simulink model "Observer_e_modello"  (R2023a)
settings: Solver=ode45  StartTime=0.0  StopTime=102  RelTol=1e-2  EnableMultiTasking=on
values from neighbouring files (symbols this model uses):
  xk0_mod = 0.9*ones(states_tot, 1)    [Convergence_observer.m]
  xk0_obs = 0*ones(states_tot, 1)    [Convergence_observer.m]
  yk2_0 = 0.5*ones(4,1)    [Convergence_observer.m]
  yk6_0 = 0.5*ones(4,1)    [Convergence_observer.m]
undefined symbols (not defined in the file or in its folder): F0A, R1, R2, R3
settings Model: Creator=scattolini  LastModifiedBy=laura
settings SolverCC: AlgebraicLoopSolver=TrustRegion
settings DataIOCC: LimitDataPoints=on  SaveFormat=Array  SignalLoggingSaveFormat=ModelDataLogs  ReturnWorkspaceOutputs=off
settings OptimizationCC: BlockReduction=off  DefaultParameterBehavior=Inlined  InlineInvariantSignals=on  BufferReuse=off  ExpressionDepthLimit=2147483647  InitFltsAndDblsToZero=on  LifeSpan=inf
settings DebuggingCC: SaveWithParameterizedLinksMsg=none  UnderspecifiedInitializationDetection=Classic  MergeDetectMultiDrivingBlocksExec=none  SignalResolutionControl=TryResolveAllWithWarning  SolverPrmCheckMsg=warning  MultiTaskDSMMsg=warning  MultiTaskCondExecSysMsg=none  FcnCallInpInsideContextMsg=warning  UnconnectedInputMsg=warning  UnconnectedOutputMsg=warning  UnconnectedLineMsg=warning  StateNameClashWarn=warning  SFUnexpectedBacktrackingDiag=warning  SFNoUnconditionalDefaultTransitionDiag=warning  SFExecutionAtInitializationDiag=none  ArithmeticOperatorsInVariantConditions=warning
settings HardwareCC: ProdBitPerPointer=32  ProdBitPerSizeT=32  ProdBitPerPtrDiffT=32  ProdLargestAtomicFloat=None  ProdIntDivRoundTo=Undefined  ProdEndianess=Unspecified  ProdWordSize=32  ProdHWDeviceType=32-bit Generic
settings ModelReferenceCC: EnableRefExpFcnMdlSchedulingChecks=on  PropagateSignalLabelsOutOfModel=off
settings RTWCC: DLArmComputeVersion=19.05
settings CodeAppCC: StateflowObjectComments=on
settings GRTTargetCC: TargetFcnLib=ansi_tfl_tmw.mat  TargetLangStandard=C89/C90 (ANSI)  CombineOutputUpdateFcns=off  GRTInterface=on
settings ConfigComp: CovMetricSettings=dw  CovSaveCumulativeToWorkspaceVar=on  CovSaveSingleToWorkspaceVar=on

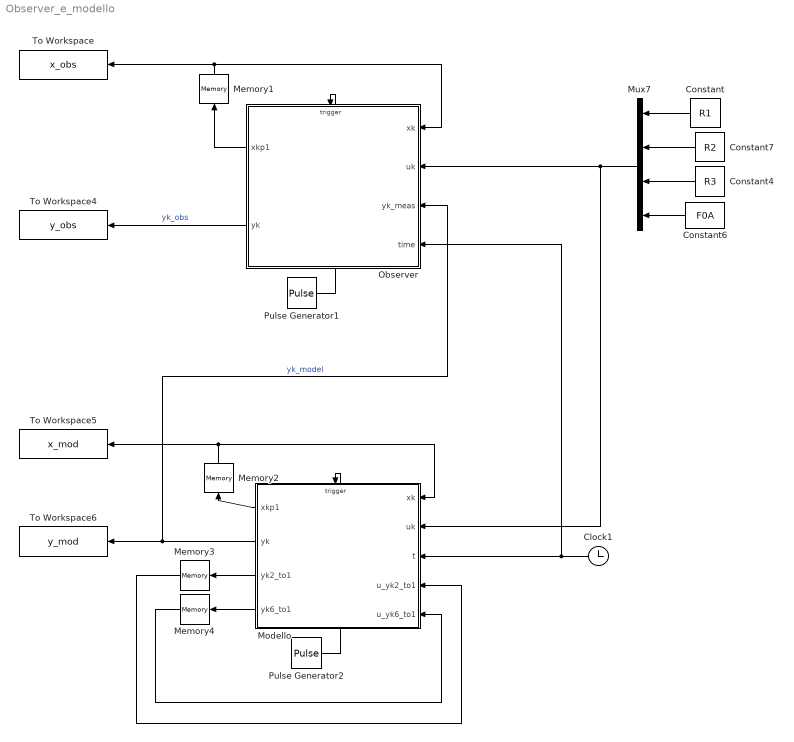
== system Observer_e_modello ==
  Clock1 : Clock
  Constant : Constant  Value=R1
  Constant4 : Constant  Value=R3
  Constant6 : Constant  Value=F0A
  Constant7 : Constant  Value=R2
  Memory1 : Memory  InitialCondition=xk0_obs
  Memory2 : Memory  InitialCondition=xk0_mod
  Memory3 : Memory  InitialCondition=yk2_0
  Memory4 : Memory  InitialCondition=yk6_0
  "Modello " : Subsystem  TreatAsAtomicUnit=on
  Mux7 : Mux
  Observer : Subsystem  TreatAsAtomicUnit=on
  Pulse Generator1 : DiscretePulseGenerator  PulseType=Time based  Period=1  PulseWidth=5
  Pulse Generator2 : DiscretePulseGenerator  PulseType=Time based  Period=1  PulseWidth=5
  To Workspace : ToWorkspace  VariableName=x_obs  SampleTime=1
  To Workspace4 : ToWorkspace  VariableName=y_obs  SampleTime=1
  To Workspace5 : ToWorkspace  VariableName=x_mod  SampleTime=1
  To Workspace6 : ToWorkspace  VariableName=y_mod  SampleTime=1
  wires:
  Pulse Generator1/1 -> Observer/Trigger
  Observer/1(xkp1) -> Memory1/1
  Memory1/1 -> Observer/1(xk), To Workspace/1
  Observer/2(yk) -> To Workspace4/1  "yk_obs"
  Mux7/1 -> Observer/2(uk), "Modello "/2(uk)
  Constant6/1 -> Mux7/4
  Clock1/1 -> Observer/4(time), "Modello "/3(t)
  "Modello "/1(xkp1) -> Memory2/1
  "Modello "/2(yk) -> Observer/3(yk_meas), To Workspace6/1  "yk_model"
  Memory2/1 -> "Modello "/1(xk), To Workspace5/1
  Pulse Generator2/1 -> "Modello "/Trigger
  "Modello "/3(yk2_to1) -> Memory3/1
  Memory3/1 -> "Modello "/4(u_yk2_to1)
  "Modello "/4(yk6_to1) -> Memory4/1
  Memory4/1 -> "Modello "/5(u_yk6_to1)
  Constant/1 -> Mux7/1
  Constant7/1 -> Mux7/2
  Constant4/1 -> Mux7/3

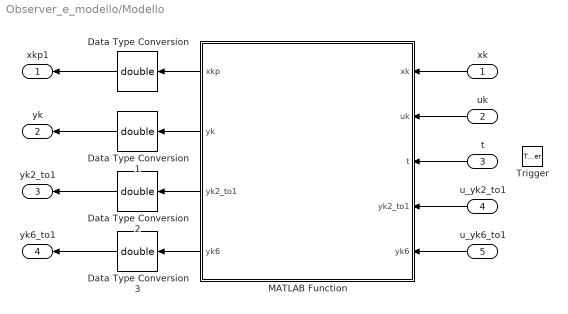
== system Observer_e_modello/Modello  ==
  xk : Inport
  uk : Inport  Port=2
  t : Inport  Port=3
  u_yk2_to1 : Inport  Port=4
  u_yk6_to1 : Inport  Port=5
  Trigger : TriggerPort  VariantControl=(inherit)
  Data Type Conversion{,1..3} (4 alike) : DataTypeConversion  OutDataTypeStr=double  RndMeth=Nearest  SaturateOnIntegerOverflow=off
  MATLAB Function : MATLAB Function  TreatAsAtomicUnit=on
  xkp1 : Outport
  yk : Outport  Port=2
  yk2_to1 : Outport  Port=3
  yk6_to1 : Outport  Port=4
  wires:
  xk/1 -> MATLAB Function/1(xk)
  MATLAB Function/2(yk) -> Data Type Conversion1/1
  MATLAB Function/1(xkp) -> Data Type Conversion/1
  Data Type Conversion/1 -> xkp1/1
  Data Type Conversion1/1 -> yk/1
  uk/1 -> MATLAB Function/2(uk)
  t/1 -> MATLAB Function/3(t)
  Data Type Conversion2/1 -> yk2_to1/1
  MATLAB Function/3(yk2_to1) -> Data Type Conversion2/1
  Data Type Conversion3/1 -> yk6_to1/1
  MATLAB Function/4(yk6) -> Data Type Conversion3/1
  u_yk6_to1/1 -> MATLAB Function/5("yk6 ")
  u_yk2_to1/1 -> MATLAB Function/4("yk2_to1 ")

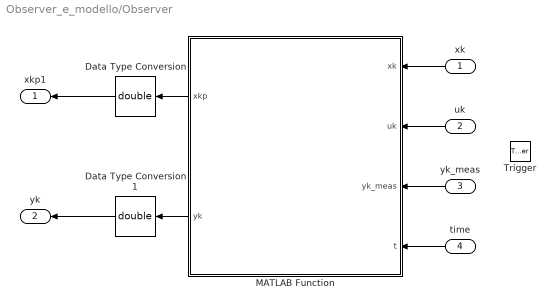
== system Observer_e_modello/Observer ==
  xk : Inport
  uk : Inport  Port=2
  yk_meas : Inport  Port=3
  time : Inport  Port=4
  Trigger : TriggerPort  VariantControl=(inherit)
  Data Type Conversion : DataTypeConversion  OutDataTypeStr=double  RndMeth=Nearest  SaturateOnIntegerOverflow=off
  Data Type Conversion1 : DataTypeConversion  OutDataTypeStr=double  RndMeth=Nearest  SaturateOnIntegerOverflow=off
  MATLAB Function : MATLAB Function  TreatAsAtomicUnit=on
  xkp1 : Outport
  yk : Outport  Port=2
  wires:
  xk/1 -> MATLAB Function/1(xk)
  uk/1 -> MATLAB Function/2(uk)
  MATLAB Function/2(yk) -> Data Type Conversion1/1
  MATLAB Function/1(xkp) -> Data Type Conversion/1
  Data Type Conversion/1 -> xkp1/1
  Data Type Conversion1/1 -> yk/1
  yk_meas/1 -> MATLAB Function/3(yk_meas)
  time/1 -> MATLAB Function/4(t)

== matlab function Observer_e_modello/Observer/MATLAB Function ==
  data: xkp output; xk input; uk input; yk_meas input; t input; yk output
function [xkp, yk] = RNN(xk, uk, yk_meas, t)

    if t <= 1
        xk = 0*ones(18, 1);
    end

    n_states = [3,3,3,3,3,3];
    layers_file = load("layers_file.mat");
    layers_file = layers_file.layers_file;
    input_scaler_bias = load("input_scaler_bias.mat");
    input_scaler_scale_common = load("input_scaler_scale_common.mat");
    output_scaler_bias = load("output_scaler_bias.mat");
    output_scaler_scale_common = load("output_scaler_scale_common.mat");
    
    % Best observer weight
    Lz1_sol = load("Lz1_sol.mat");
    Lf1_sol = load("Lf1_sol.mat");
    Lz1 = Lz1_sol.Lz1;
    Lf1 = Lf1_sol.Lf1;
    Lz2_sol = load("Lz2_sol.mat");
    Lf2_sol = load("Lf2_sol.mat");
    Lz2 = Lz2_sol.Lz2;
    Lf2 = Lf2_sol.Lf2;
    Lz3_sol = load("Lz3_sol.mat");
    Lf3_sol = load("Lf3_sol.mat");
    Lz3 = Lz3_sol.Lz3;
    Lf3 = Lf3_sol.Lf3;
    Lz4_sol = load("Lz4_sol.mat");
    Lf4_sol = load("Lf4_sol.mat");
    Lz4 = Lz4_sol.Lz4;
    Lf4 = Lf4_sol.Lf4;
    Lz5_sol = load("Lz5_sol.mat");
    Lf5_sol = load("Lf5_sol.mat");
    Lz5 = Lz5_sol.Lz5;
    Lf5 = Lf5_sol.Lf5;
    Lz6_sol = load("Lz6_sol.mat");
    Lf6_sol = load("Lf6_sol.mat");
    Lz6 = Lz6_sol.Lz6;
    Lf6 = Lf6_sol.Lf6;

    % Scale input and output
    uk = (uk  - (input_scaler_bias.input_scaler_bias).') ./ (input_scaler_scale_common.input_scaler_scale_common).';
    %yk_meas = [yk_meas(1)*yk_meas(2); yk_meas(1)*yk_meas(3); yk_meas(1)*yk_meas(4); yk_meas(1)*yk_meas(5); yk_meas(6)*yk_meas(7); yk_meas(6)*yk_meas(8); yk_meas(6)*yk_meas(9); yk_meas(6)*yk_meas(10); yk_meas(11)*yk_meas(12); yk_meas(11)*yk_meas(13); yk_meas(11)*yk_meas(14); yk_meas(11)*yk_meas(15); yk_meas(16)*yk_meas(17); yk_meas(11)*yk_meas(18); yk_meas(11)*yk_meas(19); yk_meas(11)*yk_meas(20); yk_meas(21)*yk_meas(22); yk_meas(21)*yk_meas(23); yk_meas(21)*yk_meas(24); yk_meas(21)*yk_meas(25); yk_meas(26)*yk_meas(27); yk_meas(26)*yk_meas(28); yk_meas(26)*yk_meas(29); yk_meas(26)*yk_meas(30); yk_meas(31)*yk_meas(32); yk_meas(31)*yk_meas(33); yk_meas(31)*yk_meas(34); yk_meas(31)*yk_meas(35)];
    yk_meas = (yk_meas  - (output_scaler_bias.output_scaler_bias).') ./ (output_scaler_scale_common.output_scaler_scale_common).';

    % GRU 1
    yk1_meas = yk_meas(1:4,:);
    yk2_to1_meas = yk_meas(5:8,:);
    yk6_meas = yk_meas(25:28,:);
    uk1 = [uk(1,:); uk(3:4,:); yk2_to1_meas; yk6_meas];
    xk1 = xk(1:n_states(1),:);    
    yk1 = layers_file.layers{1,2}.weights.weight * xk1 + (layers_file.layers{1,2}.weights.bias).';
    zk1 = sigmoidfunction((layers_file.layers{1,1}.weights.Wzf(:,1:n_states(1))).' * uk1 + (layers_file.layers{1,1}.weights.Uzf(:,1:n_states(1))).' * xk1 + (layers_file.layers{1,1}.weights.bzf(:,1:n_states(1))).' + Lz1*(yk1_meas-yk1) );
    fk1 = sigmoidfunction((layers_file.layers{1,1}.weights.Wzf(:,n_states(1)+1:end)).' * uk1 + (layers_file.layers{1,1}.weights.Uzf(:,n_states(1)+1:end)).' * xk1 + (layers_file.layers{1,1}.weights.bzf(:,n_states(1)+1:end)).' + Lf1*(yk1_meas-yk1) );
    phi1 = tanh((layers_file.layers{1,1}.weights.Wr).' * uk1 + (layers_file.layers{1,1}.weights.Ur).' * (fk1.* xk1) + (layers_file.layers{1,1}.weights.br).');
    xkp1 = zk1 .* xk1 + (1-zk1) .* phi1;
    
    % GRU 2    
    yk2_meas = yk_meas(5:12,:);
    yk2_to3_meas = yk_meas(9:12,:);
    uk2 = [uk(1,:); uk(3:4,:); yk1_meas];
    xk2 = xk(n_states(1)+1:n_states(1)+n_states(2),:);
    yk2 = layers_file.layers{1,4}.weights.weight * xk2 + (layers_file.layers{1,4}.weights.bias).';
    zk2 = sigmoidfunction((layers_file.layers{1,3}.weights.Wzf(:,1:n_states(2))).' * uk2 + (layers_file.layers{1,3}.weights.Uzf(:,1:n_states(2))).' * xk2 + (layers_file.layers{1,3}.weights.bzf(:,1:n_states(2))).' + Lz2*(yk2_meas-yk2) );
    fk2 = sigmoidfunction((layers_file.layers{1,3}.weights.Wzf(:,n_states(2)+1:end)).' * uk2 + (layers_file.layers{1,3}.weights.Uzf(:,n_states(2)+1:end)).' * xk2 + (layers_file.layers{1,3}.weights.bzf(:,n_states(2)+1:end)).' + Lf2*(yk2_meas-yk2) );
    phi2 = tanh((layers_file.layers{1,3}.weights.Wr).' * uk2 + (layers_file.layers{1,3}.weights.Ur).' * (fk2.* xk2) + (layers_file.layers{1,3}.weights.br).');
    xkp2 = zk2 .* xk2 + (1-zk2) .* phi2;
    
    % GRU 3
    yk3_meas = yk_meas(13:16,:);
    uk3 = [uk(2:4,:); yk2_to3_meas];
    xk3 = xk(n_states(1)+n_states(2)+1:n_states(1)+n_states(2)+n_states(3),:);
    yk3 = layers_file.layers{1,6}.weights.weight * xk3 + (layers_file.layers{1,6}.weights.bias).';
    zk3 = sigmoidfunction((layers_file.layers{1,5}.weights.Wzf(:,1:n_states(3))).' * uk3 + (layers_file.layers{1,5}.weights.Uzf(:,1:n_states(3))).' * xk3 + (layers_file.layers{1,5}.weights.bzf(:,1:n_states(3))).' + Lz3*(yk3_meas-yk3) );
    fk3 = sigmoidfunction((layers_file.layers{1,5}.weights.Wzf(:,n_states(3)+1:end)).' * uk3 + (layers_file.layers{1,5}.weights.Uzf(:,n_states(3)+1:end)).' * xk3 + (layers_file.layers{1,5}.weights.bzf(:,n_states(3)+1:end)).' + Lf3*(yk3_meas-yk3) );
    phi3 = tanh((layers_file.layers{1,5}.weights.Wr).' * uk3 + (layers_file.layers{1,5}.weights.Ur).' * (fk3.* xk3) + (layers_file.layers{1,5}.weights.br).');
    xkp3 = zk3 .* xk3 + (1-zk3) .* phi3;

    % GRU 4
    yk4_meas = yk_meas(17:20,:);
    uk4 = [uk(2:4,:); yk3_meas];
    xk4 = xk(n_states(1)+n_states(2)+n_states(3)+1:n_states(1)+n_states(2)+n_states(3)+n_states(4),:);
    yk4 = layers_file.layers{1,8}.weights.weight * xk4 + (layers_file.layers{1,8}.weights.bias).';
    zk4 = sigmoidfunction((layers_file.layers{1,7}.weights.Wzf(:,1:n_states(4))).' * uk4 + (layers_file.layers{1,7}.weights.Uzf(:,1:n_states(4))).' * xk4 + (layers_file.layers{1,7}.weights.bzf(:,1:n_states(4))).' + Lz4*(yk4_meas-yk4) );
    fk4 = sigmoidfunction((layers_file.layers{1,7}.weights.Wzf(:,n_states(4)+1:end)).' * uk4 + (layers_file.layers{1,7}.weights.Uzf(:,n_states(4)+1:end)).' * xk4 + (layers_file.layers{1,7}.weights.bzf(:,n_states(4)+1:end)).' + Lf4*(yk4_meas-yk4) );
    phi4 = tanh((layers_file.layers{1,7}.weights.Wr).' * uk4 + (layers_file.layers{1,7}.weights.Ur).' * (fk4.* xk4) + (layers_file.layers{1,7}.weights.br).');
    xkp4 = zk4 .* xk4 + (1-zk4) .* phi4;

    % GRU 5
    yk5_meas = yk_meas(21:24,:);
    uk5 = [uk(2:4,:); yk4_meas];
    xk5 = xk(n_states(1)+n_states(2)+n_states(3)+n_states(4)+1:n_states(1)+n_states(2)+n_states(3)+n_states(4)+n_states(5),:);
    yk5 = layers_file.layers{1,10}.weights.weight * xk5 + (layers_file.layers{1,10}.weights.bias).';
    zk5 = sigmoidfunction((layers_file.layers{1,9}.weights.Wzf(:,1:n_states(5))).' * uk5 + (layers_file.layers{1,9}.weights.Uzf(:,1:n_states(5))).' * xk5 + (layers_file.layers{1,9}.weights.bzf(:,1:n_states(5))).' + Lz5*(yk5_meas-yk5) );
    fk5 = sigmoidfunction((layers_file.layers{1,9}.weights.Wzf(:,n_states(5)+1:end)).' * uk5 + (layers_file.layers{1,9}.weights.Uzf(:,n_states(5)+1:end)).' * xk5 + (layers_file.layers{1,9}.weights.bzf(:,n_states(5)+1:end)).' + Lf5*(yk5_meas-yk5) );
    phi5 = tanh((layers_file.layers{1,9}.weights.Wr).' * uk5 + (layers_file.layers{1,9}.weights.Ur).' * (fk5.* xk5) + (layers_file.layers{1,9}.weights.br).');
    xkp5 = zk5 .* xk5 + (1-zk5) .* phi5;

    % GRU 6
    uk6 = [uk(2:4,:); yk5_meas];
    xk6 = xk(n_states(1)+n_states(2)+n_states(3)+n_states(4)+n_states(5)+1:n_states(1)+n_states(2)+n_states(3)+n_states(4)+n_states(5)+n_states(6),:);
    yk6 = layers_file.layers{1,12}.weights.weight * xk6 + (layers_file.layers{1,12}.weights.bias).';
    zk6 = sigmoidfunction((layers_file.layers{1,11}.weights.Wzf(:,1:n_states(6))).' * uk6 + (layers_file.layers{1,11}.weights.Uzf(:,1:n_states(6))).' * xk6 + (layers_file.layers{1,11}.weights.bzf(:,1:n_states(6))).' + Lz6*(yk6_meas-yk6) );
    fk6 = sigmoidfunction((layers_file.layers{1,11}.weights.Wzf(:,n_states(6)+1:end)).' * uk6 + (layers_file.layers{1,11}.weights.Uzf(:,n_states(6)+1:end)).' * xk6 + (layers_file.layers{1,11}.weights.bzf(:,n_states(6)+1:end)).' + Lf6*(yk6_meas-yk6) );
    phi6 = tanh((layers_file.layers{1,11}.weights.Wr).' * uk6 + (layers_file.layers{1,11}.weights.Ur).' * (fk6.* xk6) + (layers_file.layers{1,11}.weights.br).');
    xkp6 = zk6 .* xk6 + (1-zk6) .* phi6;
    
    % Overall
    xkp = [xkp1; xkp2; xkp3; xkp4; xkp5; xkp6];
    yk = [yk1; yk2; yk3; yk4; yk5; yk6];
    yk = yk .* (output_scaler_scale_common.output_scaler_scale_common).' + (output_scaler_bias.output_scaler_bias).';
end

== matlab function Observer_e_modello/Modello /MATLAB Function ==
  data: xkp output; xk input; uk input; t input; yk output; yk2_to1 output; yk6 output; yk2_to1 input; yk6 input
function [xkp, yk, yk2_to1, yk6] = RNN(xk, uk, t, yk2_to1, yk6)

    if t <= 1
        xk = 0.9*ones(18, 1);
    end

    n_states = [3,3,3,3,3,3];
    layers_file = load("layers_file.mat");
    layers_file = layers_file.layers_file;
    input_scaler_bias = load("input_scaler_bias.mat");
    input_scaler_scale_common = load("input_scaler_scale_common.mat");
    output_scaler_bias = load("output_scaler_bias.mat");
    output_scaler_scale_common = load("output_scaler_scale_common.mat");

    % Scale input and output
    uk = (uk  - (input_scaler_bias.input_scaler_bias).') ./ (input_scaler_scale_common.input_scaler_scale_common).';

    % GRU 1
    uk1 = [uk(1,:); uk(3:4,:); yk2_to1; yk6];
    xk1 = xk(1:n_states(1),:); 
    zk1 = sigmoidfunction((layers_file.layers{1,1}.weights.Wzf(:,1:n_states(1))).' * uk1 + (layers_file.layers{1,1}.weights.Uzf(:,1:n_states(1))).' * xk1 + (layers_file.layers{1,1}.weights.bzf(:,1:n_states(1))).');
    fk1 = sigmoidfunction((layers_file.layers{1,1}.weights.Wzf(:,n_states(1)+1:end)).' * uk1 + (layers_file.layers{1,1}.weights.Uzf(:,n_states(1)+1:end)).' * xk1 + (layers_file.layers{1,1}.weights.bzf(:,n_states(1)+1:end)).');
    phi1 = tanh((layers_file.layers{1,1}.weights.Wr).' * uk1 + (layers_file.layers{1,1}.weights.Ur).' * (fk1.* xk1) + (layers_file.layers{1,1}.weights.br).');
    xkp1 = zk1 .* xk1 + (1-zk1) .* phi1;
    yk1 = layers_file.layers{1,2}.weights.weight * xk1 + (layers_file.layers{1,2}.weights.bias).';
    
    % GRU 2
    uk2 = [uk(1,:); uk(3:4,:); yk1];
    xk2 = xk(n_states(1)+1:n_states(1)+n_states(2),:);
    zk2 = sigmoidfunction((layers_file.layers{1,3}.weights.Wzf(:,1:n_states(2))).' * uk2 + (layers_file.layers{1,3}.weights.Uzf(:,1:n_states(2))).' * xk2 + (layers_file.layers{1,3}.weights.bzf(:,1:n_states(2))).');
    fk2 = sigmoidfunction((layers_file.layers{1,3}.weights.Wzf(:,n_states(2)+1:end)).' * uk2 + (layers_file.layers{1,3}.weights.Uzf(:,n_states(2)+1:end)).' * xk2 + (layers_file.layers{1,3}.weights.bzf(:,n_states(2)+1:end)).');
    phi2 = tanh((layers_file.layers{1,3}.weights.Wr).' * uk2 + (layers_file.layers{1,3}.weights.Ur).' * (fk2.* xk2) + (layers_file.layers{1,3}.weights.br).');
    xkp2 = zk2 .* xk2 + (1-zk2) .* phi2;
    yk2 = layers_file.layers{1,4}.weights.weight * xk2 + (layers_file.layers{1,4}.weights.bias).';
    yk2_to1 = yk2(1:4,:);
    yk2_to3 = yk2(5:8,:); 
     
    % GRU 3
    uk3 = [uk(2:4,:); yk2_to3];
    xk3 = xk(n_states(1)+n_states(2)+1:n_states(1)+n_states(2)+n_states(3),:);
    zk3 = sigmoidfunction((layers_file.layers{1,5}.weights.Wzf(:,1:n_states(3))).' * uk3 + (layers_file.layers{1,5}.weights.Uzf(:,1:n_states(3))).' * xk3 + (layers_file.layers{1,5}.weights.bzf(:,1:n_states(3))).');
    fk3 = sigmoidfunction((layers_file.layers{1,5}.weights.Wzf(:,n_states(3)+1:end)).' * uk3 + (layers_file.layers{1,5}.weights.Uzf(:,n_states(3)+1:end)).' * xk3 + (layers_file.layers{1,5}.weights.bzf(:,n_states(3)+1:end)).');
    phi3 = tanh((layers_file.layers{1,5}.weights.Wr).' * uk3 + (layers_file.layers{1,5}.weights.Ur).' * (fk3.* xk3) + (layers_file.layers{1,5}.weights.br).');
    xkp3 = zk3 .* xk3 + (1-zk3) .* phi3;
    yk3 = layers_file.layers{1,6}.weights.weight * xk3 + (layers_file.layers{1,6}.weights.bias).';

    % GRU 4
    uk4 = [uk(2:4,:); yk3];
    xk4 = xk(n_states(1)+n_states(2)+n_states(3)+1:n_states(1)+n_states(2)+n_states(3)+n_states(4),:);
    zk4 = sigmoidfunction((layers_file.layers{1,7}.weights.Wzf(:,1:n_states(4))).' * uk4 + (layers_file.layers{1,7}.weights.Uzf(:,1:n_states(4))).' * xk4 + (layers_file.layers{1,7}.weights.bzf(:,1:n_states(4))).');
    fk4 = sigmoidfunction((layers_file.layers{1,7}.weights.Wzf(:,n_states(4)+1:end)).' * uk4 + (layers_file.layers{1,7}.weights.Uzf(:,n_states(4)+1:end)).' * xk4 + (layers_file.layers{1,7}.weights.bzf(:,n_states(4)+1:end)).');
    phi4 = tanh((layers_file.layers{1,7}.weights.Wr).' * uk4 + (layers_file.layers{1,7}.weights.Ur).' * (fk4.* xk4) + (layers_file.layers{1,7}.weights.br).');
    xkp4 = zk4 .* xk4 + (1-zk4) .* phi4;
    yk4 = layers_file.layers{1,8}.weights.weight * xk4 + (layers_file.layers{1,8}.weights.bias).';
    
    % GRU 5
    uk5 = [uk(2:4,:); yk4];
    xk5 = xk(n_states(1)+n_states(2)+n_states(3)+n_states(4)+1:n_states(1)+n_states(2)+n_states(3)+n_states(4)+n_states(5),:);
    zk5 = sigmoidfunction((layers_file.layers{1,9}.weights.Wzf(:,1:n_states(5))).' * uk5 + (layers_file.layers{1,9}.weights.Uzf(:,1:n_states(5))).' * xk5 + (layers_file.layers{1,9}.weights.bzf(:,1:n_states(5))).');
    fk5 = sigmoidfunction((layers_file.layers{1,9}.weights.Wzf(:,n_states(5)+1:end)).' * uk5 + (layers_file.layers{1,9}.weights.Uzf(:,n_states(5)+1:end)).' * xk5 + (layers_file.layers{1,9}.weights.bzf(:,n_states(5)+1:end)).');
    phi5 = tanh((layers_file.layers{1,9}.weights.Wr).' * uk5 + (layers_file.layers{1,9}.weights.Ur).' * (fk5.* xk5) + (layers_file.layers{1,9}.weights.br).');
    xkp5 = zk5 .* xk5 + (1-zk5) .* phi5;
    yk5 = layers_file.layers{1,10}.weights.weight * xk5 + (layers_file.layers{1,10}.weights.bias).';
    
    % GRU 6
    uk6 = [uk(2:4,:); yk5];
    xk6 = xk(n_states(1)+n_states(2)+n_states(3)+n_states(4)+n_states(5)+1:n_states(1)+n_states(2)+n_states(3)+n_states(4)+n_states(5)+n_states(6),:);
    zk6 = sigmoidfunction((layers_file.layers{1,11}.weights.Wzf(:,1:n_states(6))).' * uk6 + (layers_file.layers{1,11}.weights.Uzf(:,1:n_states(6))).' * xk6 + (layers_file.layers{1,11}.weights.bzf(:,1:n_states(6))).');
    fk6 = sigmoidfunction((layers_file.layers{1,11}.weights.Wzf(:,n_states(6)+1:end)).' * uk6 + (layers_file.layers{1,11}.weights.Uzf(:,n_states(6)+1:end)).' * xk6 + (layers_file.layers{1,11}.weights.bzf(:,n_states(6)+1:end)).');
    phi6 = tanh((layers_file.layers{1,11}.weights.Wr).' * uk6 + (layers_file.layers{1,11}.weights.Ur).' * (fk6.* xk6) + (layers_file.layers{1,11}.weights.br).');
    xkp6 = zk6 .* xk6 + (1-zk6) .* phi6;
    yk6 = layers_file.layers{1,12}.weights.weight * xk6 + (layers_file.layers{1,12}.weights.bias).';

    % Overall
    xkp = [xkp1; xkp2; xkp3; xkp4; xkp5; xkp6];
    yk = [yk1; yk2; yk3; yk4; yk5; yk6];
    yk = yk .* (output_scaler_scale_common.output_scaler_scale_common).' + (output_scaler_bias.output_scaler_bias).';
end
